simulink model "simACC"  (R2018b)
settings: Solver=VariableStepAuto  StartTime=0.0  StopTime=8  RelTol=1e-3
undefined symbols (not defined in the file or in its folder): DiscIntNeverNeededParam, Discrete, Time
libraries: libslotcar x9, simulink x4, ctrlSharedLib x3, libcontrol x1
settings Model: Creator=Lenovo  LastModifiedBy=Lenovo

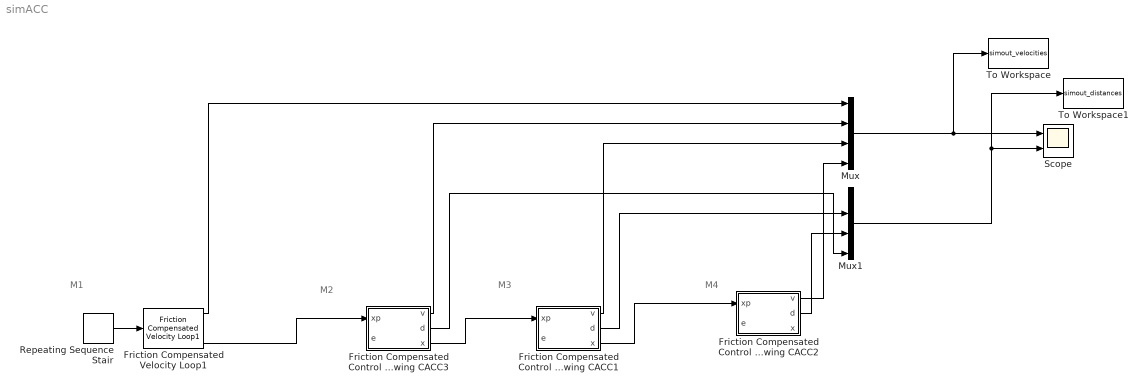
== system simACC ==
  note: M1
  note: M4
  note: M3
  note: M2
  Friction Compensated Control Effort Following CACC1 : Subsystem  AncestorBlock="libcontrol/Friction Compensated  Control Effort Following CACC1"
  Friction Compensated Control Effort Following CACC2 : Subsystem  AncestorBlock="libcontrol/Friction Compensated  Control Effort Following CACC1"
  Friction Compensated Control Effort Following CACC3 : Subsystem  AncestorBlock="libcontrol/Friction Compensated  Control Effort Following CACC1"
  Friction Compensated Velocity Loop1 : libcontrol/Friction Compensated Velocity Loop1  SystemSampleTime=-1
  Mux : Mux
  Mux1 : Mux
  Repeating Sequence Stair : simulink/Sources/Repeating Sequence Stair  OutValues=[0.8 0.5 0.8].'  tsamp=3  OutMin=[]  OutMax=[]  OutDataTypeStr=double  OutputDataTypeScalingMode=double  OutDataType=fixdt(0,8)  ConRadixGroup=Best Precision: Vector-wise  OutScaling=2^-12
  Scope : Scope  NumInputPorts=2
  To Workspace : ToWorkspace  VariableName=simout_velocities  SaveFormat=Timeseries  SampleTime=-1
  To Workspace1 : ToWorkspace  VariableName=simout_distances  SaveFormat=Timeseries  SampleTime=-1
  wires:
  Friction Compensated Control Effort Following CACC2/2(d) -> Mux1/4
  Friction Compensated Control Effort Following CACC1/2(d) -> Mux1/3
  Mux1/1 -> To Workspace1/1, Scope/2
  Friction Compensated Control Effort Following CACC3/2(d) -> Mux1/2
  Friction Compensated Control Effort Following CACC3/3(x) -> Friction Compensated Control Effort Following CACC1/1(xp)
  Friction Compensated Control Effort Following CACC1/3(x) -> Friction Compensated Control Effort Following CACC2/1(xp)
  Friction Compensated Velocity Loop1/3 -> Friction Compensated Control Effort Following CACC3/1(xp)
  Mux/1 -> To Workspace/1, Scope/1
  Friction Compensated Velocity Loop1/1 -> Mux/1
  Friction Compensated Control Effort Following CACC1/1(v) -> Mux/3
  Friction Compensated Control Effort Following CACC3/1(v) -> Mux/2
  Friction Compensated Control Effort Following CACC2/1(v) -> Mux/4
  Repeating Sequence Stair/1 -> Friction Compensated Velocity Loop1/1

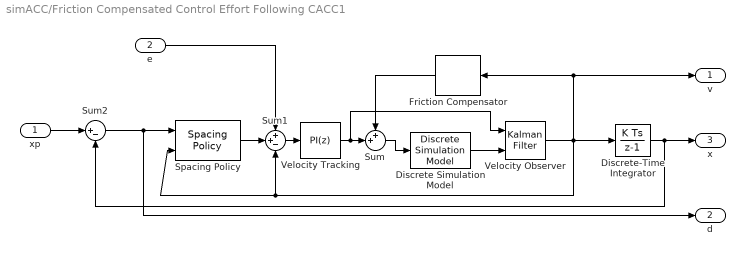
== system simACC/Friction Compensated Control Effort Following CACC1 ==
  xp : Inport
  e : Inport  Port=2
  Discrete Simulation Model : libslotcar/Discrete Simulation Model  tsparam=-1  mparam=0.173  dparam=0.018  nparam=9/28  uparam=12.25-0.7  rparam=5  kparam=0.005  ksparam=0.7183  kdparam=0.3415
  Discrete-Time Integrator : DiscreteIntegrator  InitialCondition=-0.08  SampleTime=-1  ICPrevOutput=DiscIntNeverNeededParam  ICPrevScaledInput=DiscIntNeverNeededParam
  Friction Compensator : libslotcar/Friction Compensator  coul=0.7183  visc=0.3415  Gain=1/3.9963
  Spacing Policy : libslotcar/Spacing Policy  Gain=50  dcor=0.03  h0=0.04  hv=0.1
  Sum : Sum  Inputs=++|
  Sum1 : Sum  Inputs=++-
  Sum2 : Sum  Inputs=|+-
  Velocity Observer : ctrlSharedLib/Kalman Filter  TimeDomain=Discrete-Time  UseCurrentEstimator=on  ModelSource=Individual A, B, C, D matrices  ModelSourceVariable=ss(0.95,1,1,1,0)  A=-3.46  B=23.1  C=1  D=0  NumberOfStates=1  NumberOfInputs=1  NumberOfOutputs=1  InitialEstimateSource=Dialog  X0=0  P0=10  UseK=off  UseGH=off  NumberOfProcessNoiseInputs=1  G=1  TimeInvariantG=on  H=0  TimeInvariantH=on  Q=1  TimeInvariantQ=on  R=1  TimeInvariantR=on  N=0  TimeInvariantN=on  AddInputPort=on  AddEnablePort=off  OutputEstimatedY=off  OutputP=off  Ts=1/400
      settings: SourceProductBaseCode=CT
  Velocity Tracking : simulink/Continuous/PID Controller  Controller=PI  Form=Parallel  TimeDomain=Discrete-time  SampleTime=-1  IntegratorMethod=Forward Euler  FilterMethod=Forward Euler  ControllerParametersSource=internal  P=0.202863589993018  I=2.14911342042457  D=0  UseFilter=on  N=100  TunerSelectOption=Transfer Function Based (PID Tuner App)  InitialConditionSource=internal  InitialConditionForIntegrator=0  InitialConditionForFilter=0  DifferentiatorICPrevScaledInput=0  ExternalReset=none  TrackingMode=off  Kt=1  LimitOutput=on  UpperSaturationLimit=0.4  LowerSaturationLimit=-0.4  LinearizeAsGain=off  AntiWindupMode=clamping  Kb=1  POutMin=[]  POutMax=[]  IOutMin=[]  IOutMax=[]  DOutMin=[]  DOutMax=[]  NOutMin=[]  NOutMax=[]  SumOutMin=[]  SumOutMax=[]  SaturationOutMin=[]  SaturationOutMax=[]  PParamMin=[]  PParamMax=[]  IParamMin=[]  IParamMax=[]  DParamMin=[]  DParamMax=[]  NParamMin=[]  NParamMax=[]  KbParamMin=[]  KbParamMax=[]  KtParamMin=[]  KtParamMax=[]  KbOutMin=[]  KbOutMax=[]  KtOutMin=[]  KtOutMax=[]  IntegratorOutMin=[]  IntegratorOutMax=[]  FilterOutMin=[]  FilterOutMax=[]  SumI1OutMin=[]  SumI1OutMax=[]  SumI2OutMin=[]  SumI2OutMax=[]  SumI3OutMin=[]  SumI3OutMax=[]  SumI4OutMin=[]  SumI4OutMax=[]  SumDOutMin=[]  SumDOutMax=[]  DifferentiatorOutMin=[]  DifferentiatorOutMax=[]  FilterDiffOutCoefMin=[]  FilterDiffOutCoefMax=[]  ReciprocalOutMin=[]  ReciprocalOutMax=[]  SumDenOutMin=[]  SumDenOutMax=[]  SumNumOutMin=[]  SumNumOutMax=[]  DivideOutMin=[]  DivideOutMax=[]  IntegratorContinuousStateAttributes=''  IntegratorStateMustResolveToSignalObject=off  IntegratorRTWStateStorageClass=Auto  FilterContinuousStateAttributes=''  FilterStateMustResolveToSignalObject=off  FilterRTWStateStorageClass=Auto  ParallelPVariant=InternalParameters  IdealPVariant=Disabled  IVariant=InternalParameters  DVariant=Disabled  IntegratorVariant=Discrete  SatVariant=Enabled  AWVariant=DiscClampingParallel  PCopyVariant=Disabled  TRVariant=Disabled  FdbkBlocksVariant=Forward  IdealPFdbkVariant=Disabled  SatFdbkVariant=Disabled  DerivativeFilterVariant=Disabled  NVariant=Disabled  NCopyVariant=Disabled_SignalSpec  FilterICVariant=Disabled  IntegratorICVariant=InternalICs  ExternalResetVariant=Disabled  TRSumVariant=Passthrough  SumFdbkVariant=Disabled  SumVariant=Sum_PI
  v : Outport
  d : Outport  Port=2
  x : Outport  Port=3
  wires:
  Discrete-Time Integrator/1 -> x/1, Sum2/2
  Sum2/1 -> Spacing Policy/1, d/1
  Sum/1 -> Discrete Simulation Model/1
  xp/1 -> Sum2/1
  Discrete Simulation Model/1 -> Velocity Observer/2
  Sum1/1 -> Velocity Tracking/1
  Velocity Tracking/1 -> Sum/2, Velocity Observer/1
  Velocity Observer/1 -> Discrete-Time Integrator/1, Friction Compensator/1, v/1, Spacing Policy/2, Sum1/3
  Friction Compensator/1 -> Sum/1
  Spacing Policy/1 -> Sum1/2
  e/1 -> Sum1/1

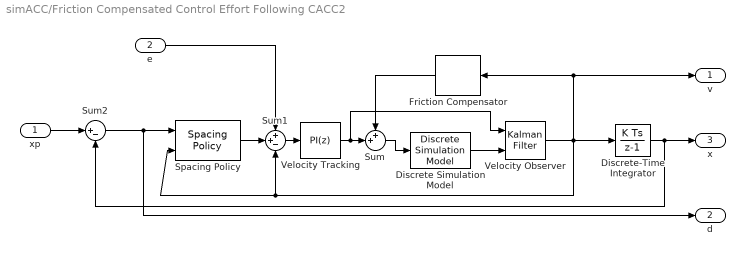
== system simACC/Friction Compensated Control Effort Following CACC2 ==
  xp : Inport
  e : Inport  Port=2
  Discrete Simulation Model : libslotcar/Discrete Simulation Model  tsparam=-1  mparam=0.173  dparam=0.018  nparam=9/28  uparam=12.25-0.7  rparam=5  kparam=0.005  ksparam=0.7183  kdparam=0.3415
  Discrete-Time Integrator : DiscreteIntegrator  InitialCondition=-0.12  SampleTime=-1  ICPrevOutput=DiscIntNeverNeededParam  ICPrevScaledInput=DiscIntNeverNeededParam
  Friction Compensator : libslotcar/Friction Compensator  coul=0.7183  visc=0.3415  Gain=1/3.9963
  Spacing Policy : libslotcar/Spacing Policy  Gain=50  dcor=0.03  h0=0.04  hv=0.1
  Sum : Sum  Inputs=++|
  Sum1 : Sum  Inputs=++-
  Sum2 : Sum  Inputs=|+-
  Velocity Observer : ctrlSharedLib/Kalman Filter  TimeDomain=Discrete-Time  UseCurrentEstimator=on  ModelSource=Individual A, B, C, D matrices  ModelSourceVariable=ss(0.95,1,1,1,0)  A=-3.46  B=23.1  C=1  D=0  NumberOfStates=1  NumberOfInputs=1  NumberOfOutputs=1  InitialEstimateSource=Dialog  X0=0  P0=10  UseK=off  UseGH=off  NumberOfProcessNoiseInputs=1  G=1  TimeInvariantG=on  H=0  TimeInvariantH=on  Q=1  TimeInvariantQ=on  R=1  TimeInvariantR=on  N=0  TimeInvariantN=on  AddInputPort=on  AddEnablePort=off  OutputEstimatedY=off  OutputP=off  Ts=1/400
      settings: SourceProductBaseCode=CT
  Velocity Tracking : simulink/Continuous/PID Controller  Controller=PI  Form=Parallel  TimeDomain=Discrete-time  SampleTime=-1  IntegratorMethod=Forward Euler  FilterMethod=Forward Euler  ControllerParametersSource=internal  P=0.202863589993018  I=2.14911342042457  D=0  UseFilter=on  N=100  TunerSelectOption=Transfer Function Based (PID Tuner App)  InitialConditionSource=internal  InitialConditionForIntegrator=0  InitialConditionForFilter=0  DifferentiatorICPrevScaledInput=0  ExternalReset=none  TrackingMode=off  Kt=1  LimitOutput=on  UpperSaturationLimit=0.4  LowerSaturationLimit=-0.4  LinearizeAsGain=off  AntiWindupMode=clamping  Kb=1  POutMin=[]  POutMax=[]  IOutMin=[]  IOutMax=[]  DOutMin=[]  DOutMax=[]  NOutMin=[]  NOutMax=[]  SumOutMin=[]  SumOutMax=[]  SaturationOutMin=[]  SaturationOutMax=[]  PParamMin=[]  PParamMax=[]  IParamMin=[]  IParamMax=[]  DParamMin=[]  DParamMax=[]  NParamMin=[]  NParamMax=[]  KbParamMin=[]  KbParamMax=[]  KtParamMin=[]  KtParamMax=[]  KbOutMin=[]  KbOutMax=[]  KtOutMin=[]  KtOutMax=[]  IntegratorOutMin=[]  IntegratorOutMax=[]  FilterOutMin=[]  FilterOutMax=[]  SumI1OutMin=[]  SumI1OutMax=[]  SumI2OutMin=[]  SumI2OutMax=[]  SumI3OutMin=[]  SumI3OutMax=[]  SumI4OutMin=[]  SumI4OutMax=[]  SumDOutMin=[]  SumDOutMax=[]  DifferentiatorOutMin=[]  DifferentiatorOutMax=[]  FilterDiffOutCoefMin=[]  FilterDiffOutCoefMax=[]  ReciprocalOutMin=[]  ReciprocalOutMax=[]  SumDenOutMin=[]  SumDenOutMax=[]  SumNumOutMin=[]  SumNumOutMax=[]  DivideOutMin=[]  DivideOutMax=[]  IntegratorContinuousStateAttributes=''  IntegratorStateMustResolveToSignalObject=off  IntegratorRTWStateStorageClass=Auto  FilterContinuousStateAttributes=''  FilterStateMustResolveToSignalObject=off  FilterRTWStateStorageClass=Auto  ParallelPVariant=InternalParameters  IdealPVariant=Disabled  IVariant=InternalParameters  DVariant=Disabled  IntegratorVariant=Discrete  SatVariant=Enabled  AWVariant=DiscClampingParallel  PCopyVariant=Disabled  TRVariant=Disabled  FdbkBlocksVariant=Forward  IdealPFdbkVariant=Disabled  SatFdbkVariant=Disabled  DerivativeFilterVariant=Disabled  NVariant=Disabled  NCopyVariant=Disabled_SignalSpec  FilterICVariant=Disabled  IntegratorICVariant=InternalICs  ExternalResetVariant=Disabled  TRSumVariant=Passthrough  SumFdbkVariant=Disabled  SumVariant=Sum_PI
  v : Outport
  d : Outport  Port=2
  x : Outport  Port=3
  wires:
  Discrete-Time Integrator/1 -> x/1, Sum2/2
  Sum2/1 -> Spacing Policy/1, d/1
  Sum/1 -> Discrete Simulation Model/1
  xp/1 -> Sum2/1
  Discrete Simulation Model/1 -> Velocity Observer/2
  Sum1/1 -> Velocity Tracking/1
  Velocity Tracking/1 -> Sum/2, Velocity Observer/1
  Velocity Observer/1 -> Discrete-Time Integrator/1, Friction Compensator/1, v/1, Spacing Policy/2, Sum1/3
  Friction Compensator/1 -> Sum/1
  Spacing Policy/1 -> Sum1/2
  e/1 -> Sum1/1

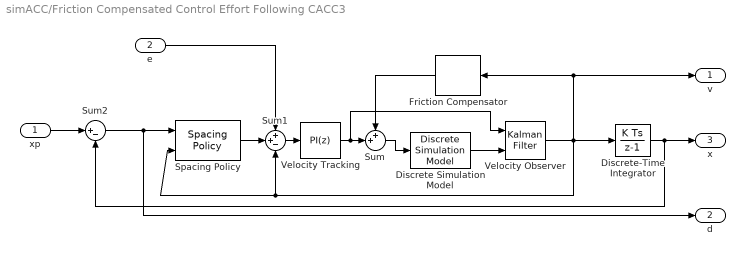
== system simACC/Friction Compensated Control Effort Following CACC3 ==
  xp : Inport
  e : Inport  Port=2
  Discrete Simulation Model : libslotcar/Discrete Simulation Model  tsparam=-1  mparam=0.173  dparam=0.018  nparam=9/28  uparam=12.25-0.7  rparam=5  kparam=0.005  ksparam=0.7183  kdparam=0.3415
  Discrete-Time Integrator : DiscreteIntegrator  InitialCondition=-0.04  SampleTime=-1  ICPrevOutput=DiscIntNeverNeededParam  ICPrevScaledInput=DiscIntNeverNeededParam
  Friction Compensator : libslotcar/Friction Compensator  coul=0.7183  visc=0.3415  Gain=1/3.9963
  Spacing Policy : libslotcar/Spacing Policy  Gain=50  dcor=0.03  h0=0.04  hv=0.1
  Sum : Sum  Inputs=++|
  Sum1 : Sum  Inputs=++-
  Sum2 : Sum  Inputs=|+-
  Velocity Observer : ctrlSharedLib/Kalman Filter  TimeDomain=Discrete-Time  UseCurrentEstimator=on  ModelSource=Individual A, B, C, D matrices  ModelSourceVariable=ss(0.95,1,1,1,0)  A=-3.46  B=23.1  C=1  D=0  NumberOfStates=1  NumberOfInputs=1  NumberOfOutputs=1  InitialEstimateSource=Dialog  X0=0  P0=10  UseK=off  UseGH=off  NumberOfProcessNoiseInputs=1  G=1  TimeInvariantG=on  H=0  TimeInvariantH=on  Q=1  TimeInvariantQ=on  R=1  TimeInvariantR=on  N=0  TimeInvariantN=on  AddInputPort=on  AddEnablePort=off  OutputEstimatedY=off  OutputP=off  Ts=1/400
      settings: SourceProductBaseCode=CT
  Velocity Tracking : simulink/Continuous/PID Controller  Controller=PI  Form=Parallel  TimeDomain=Discrete-time  SampleTime=-1  IntegratorMethod=Forward Euler  FilterMethod=Forward Euler  ControllerParametersSource=internal  P=0.202863589993018  I=2.14911342042457  D=0  UseFilter=on  N=100  TunerSelectOption=Transfer Function Based (PID Tuner App)  InitialConditionSource=internal  InitialConditionForIntegrator=0  InitialConditionForFilter=0  DifferentiatorICPrevScaledInput=0  ExternalReset=none  TrackingMode=off  Kt=1  LimitOutput=on  UpperSaturationLimit=0.4  LowerSaturationLimit=-0.4  LinearizeAsGain=off  AntiWindupMode=clamping  Kb=1  POutMin=[]  POutMax=[]  IOutMin=[]  IOutMax=[]  DOutMin=[]  DOutMax=[]  NOutMin=[]  NOutMax=[]  SumOutMin=[]  SumOutMax=[]  SaturationOutMin=[]  SaturationOutMax=[]  PParamMin=[]  PParamMax=[]  IParamMin=[]  IParamMax=[]  DParamMin=[]  DParamMax=[]  NParamMin=[]  NParamMax=[]  KbParamMin=[]  KbParamMax=[]  KtParamMin=[]  KtParamMax=[]  KbOutMin=[]  KbOutMax=[]  KtOutMin=[]  KtOutMax=[]  IntegratorOutMin=[]  IntegratorOutMax=[]  FilterOutMin=[]  FilterOutMax=[]  SumI1OutMin=[]  SumI1OutMax=[]  SumI2OutMin=[]  SumI2OutMax=[]  SumI3OutMin=[]  SumI3OutMax=[]  SumI4OutMin=[]  SumI4OutMax=[]  SumDOutMin=[]  SumDOutMax=[]  DifferentiatorOutMin=[]  DifferentiatorOutMax=[]  FilterDiffOutCoefMin=[]  FilterDiffOutCoefMax=[]  ReciprocalOutMin=[]  ReciprocalOutMax=[]  SumDenOutMin=[]  SumDenOutMax=[]  SumNumOutMin=[]  SumNumOutMax=[]  DivideOutMin=[]  DivideOutMax=[]  IntegratorContinuousStateAttributes=''  IntegratorStateMustResolveToSignalObject=off  IntegratorRTWStateStorageClass=Auto  FilterContinuousStateAttributes=''  FilterStateMustResolveToSignalObject=off  FilterRTWStateStorageClass=Auto  ParallelPVariant=InternalParameters  IdealPVariant=Disabled  IVariant=InternalParameters  DVariant=Disabled  IntegratorVariant=Discrete  SatVariant=Enabled  AWVariant=DiscClampingParallel  PCopyVariant=Disabled  TRVariant=Disabled  FdbkBlocksVariant=Forward  IdealPFdbkVariant=Disabled  SatFdbkVariant=Disabled  DerivativeFilterVariant=Disabled  NVariant=Disabled  NCopyVariant=Disabled_SignalSpec  FilterICVariant=Disabled  IntegratorICVariant=InternalICs  ExternalResetVariant=Disabled  TRSumVariant=Passthrough  SumFdbkVariant=Disabled  SumVariant=Sum_PI
  v : Outport
  d : Outport  Port=2
  x : Outport  Port=3
  wires:
  Discrete-Time Integrator/1 -> x/1, Sum2/2
  Sum2/1 -> Spacing Policy/1, d/1
  Sum/1 -> Discrete Simulation Model/1
  xp/1 -> Sum2/1
  Discrete Simulation Model/1 -> Velocity Observer/2
  Sum1/1 -> Velocity Tracking/1
  Velocity Tracking/1 -> Sum/2, Velocity Observer/1
  Velocity Observer/1 -> Discrete-Time Integrator/1, Friction Compensator/1, v/1, Spacing Policy/2, Sum1/3
  Friction Compensator/1 -> Sum/1
  Spacing Policy/1 -> Sum1/2
  e/1 -> Sum1/1
